simulink model "Day2"  (R2017b)
settings: Solver=VariableStepAuto  StartTime=0.0  StopTime=10.0  RelTol=1e-3
PreLoadFcn:
  | run('day2_input.m')
InitFcn:
  | run('day2_input.m')
values from neighbouring files (symbols this model uses):
  g = 9.8    [day2_input.m]    (also in day2_input.mat)
  h = 100    [day2_input.m]    (also in day2_input.mat)
  v = sqrt(v0*v0 + g*g*t*t)    [day2_input.m]
  v0 = 30    [day2_input.m]    (also in day2_input.mat)
settings Model: Creator=Admin  LastModifiedBy=Admin

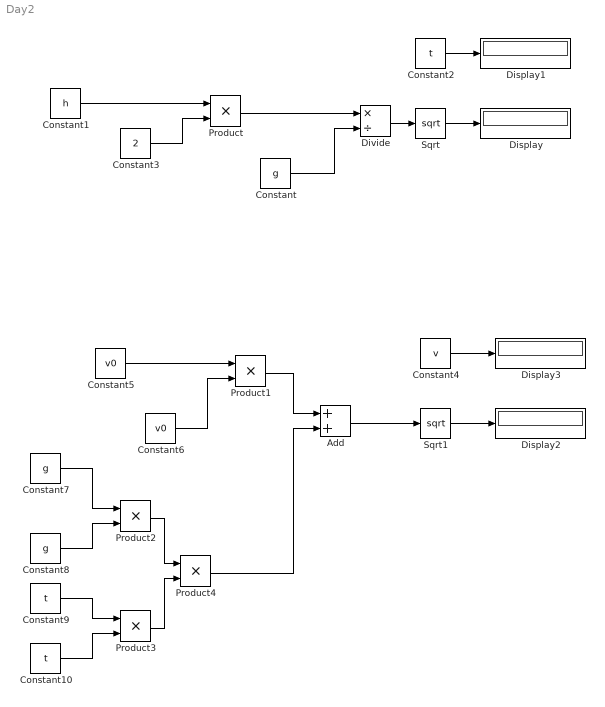
== system Day2 ==
  Add : Sum
  Constant : Constant  Value=g
  Constant1 : Constant  Value=h
  Constant10 : Constant  Value=t
  Constant2 : Constant  Value=t
  Constant3 : Constant  Value=2
  Constant4 : Constant  Value=v
  Constant5 : Constant  Value=v0
  Constant6 : Constant  Value=v0
  Constant7 : Constant  Value=g
  Constant8 : Constant  Value=g
  Constant9 : Constant  Value=t
  Display{,1..3} (4 alike) : Display
  Divide : Product  Inputs=*/
  Product{,1..4} (5 alike) : Product
  Sqrt : Sqrt  SaturateOnIntegerOverflow=on
  Sqrt1 : Sqrt  SaturateOnIntegerOverflow=on
  wires:
  Sqrt/1 -> Display/1
  Constant/1 -> Divide/2
  Constant1/1 -> Product/1
  Constant3/1 -> Product/2
  Product/1 -> Divide/1
  Divide/1 -> Sqrt/1
  Constant2/1 -> Display1/1
  Constant4/1 -> Display3/1
  Sqrt1/1 -> Display2/1
  Add/1 -> Sqrt1/1
  Constant5/1 -> Product1/1
  Constant6/1 -> Product1/2
  Constant8/1 -> Product2/2
  Constant7/1 -> Product2/1
  Constant9/1 -> Product3/1
  Constant10/1 -> Product3/2
  Product2/1 -> Product4/1
  Product3/1 -> Product4/2
  Product1/1 -> Add/1
  Product4/1 -> Add/2
